simulink model "FYP_Model_ClosedLoop"  (R2014b)
settings: Solver=ode3  StartTime=0.0  StopTime=4  FixedStep=0.0001  MaxStep=0.00001  MinStep=0.00002  RelTol=1e-3
values from neighbouring files (symbols this model uses):
  C = 2.2389314028e-09    [Example_Data.mat]    (also in calculate_constants.m = sqrt(I*K)/Q)
  Capacitance = [1.60057592274e-13 1.6356865827e-13 1.66667495448e-13 1.71350652646e-13 1.74939566926e-13 1.79103436846e-13 1.83468868499e-13 1.88053142462e-13 1.92872426544e-13 1.97945050457e-13 2.03290835825e-13 2.08663004534e-13 ... (161 elements, 1x161)]    [Example_Data.mat]    (also in SC_Transformation.m = E*(l*1e-6)*num_of_gaps)
  I = 2.138022e-10    [Example_Data.mat]    (also in calculate_constants.m = (1/12)*m*w*w)
  K = 8.44057253633e-05    [Example_Data.mat]    (also in calculate_constants.m = Wn*Wn*I)
  theta = [-7.61408173959 -7.51775010326 -7.42143983606 -7.32515065184 -7.22888226498 -7.13263439042 -7.03640674362 -6.94019904057 -6.84401099779 -6.74784233231 -6.65169276165 -6.55556200382 ... (160 elements, 1x160)]    [Example_Data.mat]    (also in SC_Transformation.m = (asin(x1/3000))*(180/pi))
  theta1 = [-7.66225566077 -7.56591323238 -7.46959231642 -7.37329262644 -7.27701387657 -7.18075578146 -7.08451805631 -6.98830041685 -6.89210257935 -6.79592426056 -6.69976517776 -6.60362504873 ... (161 elements, 1x161)]    [Example_Data.mat]    (also in SC_Transformation.m = (asin(x/3000))*(180/pi))
  TorqueN = [1.05331979874e-12 9.29651153439e-13 1.4049471593e-12 1.07667428419e-12 1.24916097602e-12 1.30962949594e-12 1.37528218875e-12 1.44578522446e-12 1.52178717406e-12 1.6037356104e-12 1.6116506126e-12 1.87151628256e-12 ... (160 elements, 1x160)]    [Example_Data.mat]    (also in SC_Transformation.m = Torque/(V*V))
  V = 60    [Example_Data.mat]    (also in SC_Transformation.m = 30; Simulink_Iterate.m = V_array(i))
libraries: simulink x7, simulink_extras x1
settings Model: Creator=Kishan  LastModifiedBy=Kishan
settings DataIOCC: SaveFormat=StructureWithTime  SaveOutput=off  ReturnWorkspaceOutputsName=yout

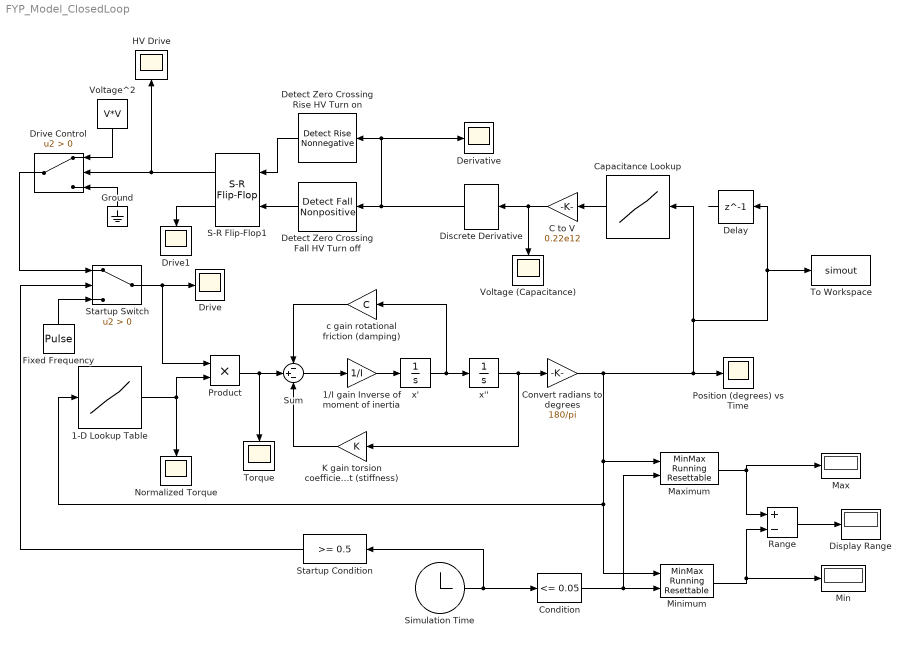
== system FYP_Model_ClosedLoop ==
  1-D Lookup Table : Lookup_n-D  NumberOfTableDimensions=1  BreakpointsForDimension1=theta  IndexSearchMethod=Linear search  Table=TorqueN  InternalRulePriority=Speed  RndMeth=Simplest  InputSameDT=on
  1/I gain Inverse of moment of inertia : Gain  Gain=1/I
  C to V : Gain  Gain=0.22e12
  Capacitance Lookup : Lookup_n-D  NumberOfTableDimensions=1  BreakpointsForDimension1=theta1  IndexSearchMethod=Linear search  Table=Capacitance  InternalRulePriority=Speed  RndMeth=Simplest  InputSameDT=on
  Condition : simulink/Logic and Bit Operations/Compare To Constant  relop=<=  const=0.05  OutDataTypeStr=boolean
  Convert radians to degrees : Gain  Gain=180/pi
  Delay : Delay  DelayLength=1  InitialCondition=0
  Derivative : Scope
      settings: TimeRange=5  YMin=0  YMax=10  SaveName=ScopeData6
  Detect Zero Crossing Fall HV Turn off : simulink/Logic and Bit Operations/Detect Fall Nonpositive  vinit=0  InputProcessing=Inherited  OutDataTypeStr=boolean
  Detect Zero Crossing Rise HV Turn on : simulink/Logic and Bit Operations/Detect Rise Nonnegative  vinit=0  InputProcessing=Inherited  OutDataTypeStr=boolean
  Discrete Derivative : simulink/Discrete/Discrete Derivative  gainval=1.0  ICPrevScaledInput=0.1  InputProcessing=Inherited  OutMin=[]  OutMax=[]  OutDataType=fixdt(1, 16)  OutScaling=2^-10  DoSatur=off
  Display Range : Display
  Drive : Scope
      settings: TimeRange=4  YMin=4.99210822998873  YMax=16.99210822998873  SaveName=ScopeData4
  Drive Control : Switch  Criteria=u2 > Threshold
  Drive1 : Scope
      settings: TimeRange=4  YMin=4.99210822998873  YMax=16.99210822998873  SaveName=ScopeData2
  Fixed Frequency : DiscretePulseGenerator  PulseType=Time based  Amplitude=V*V  Period=0.022  PulseWidth=50  SampleTime=0.0025
  Ground : Ground
  HV Drive : Scope
      settings: TimeRange=3  YMin=0  YMax=1  SaveName=ScopeData11
  K gain torsion coefficient (stiffness) : Gain  Gain=K
  Max : Display
  Maximum : simulink/Math Operations/MinMax Running Resettable  Function=max  vinit=0.0
  Min : Display
  Minimum : simulink/Math Operations/MinMax Running Resettable  Function=min  vinit=10
  Normalized Torque : Scope
      settings: TimeRange=0.009043223963749458  YMin=0  YMax=1
  Position (degrees) vs Time : Scope
      settings: TimeRange=4  YMin=-0.15  YMax=0.15
  Product : Product
  Range : Sum  Inputs=+-
  S-R Flip-Flop1 : simulink_extras/Flip Flops/S-R Flip-Flop  initial_condition=0
  Simulation Time : Clock
  Startup Condition : simulink/Logic and Bit Operations/Compare To Constant  relop=>=  const=0.5  OutDataTypeStr=uint8
  Startup Switch : Switch  Criteria=u2 > Threshold
  Sum : Sum  Inputs=-+-
  To Workspace : ToWorkspace  VariableName=simout  SaveFormat=Structure With Time  SampleTime=-1
  Torque : Scope
      settings: TimeRange=0.009043223963749458  YMin=0  YMax=1  SaveName=ScopeData3
  Voltage (Capacitance) : Scope
      settings: TimeRange=5  YMin=0  YMax=10  SaveName=ScopeData5
  Voltage^2 : Constant  Value=V*V
  c gain rotational friction (damping) : Gain  Gain=C
  x' : Integrator
  x'' : Integrator
  wires:
  x'/1 -> x''/1, c gain rotational friction (damping)/1
  1/I gain Inverse of moment of inertia/1 -> x'/1
  Sum/1 -> 1/I gain Inverse of moment of inertia/1
  K gain torsion coefficient (stiffness)/1 -> Sum/3
  c gain rotational friction (damping)/1 -> Sum/1
  1-D Lookup Table/1 -> Product/2, Normalized Torque/1
  Product/1 -> Torque/1, Sum/2
  x''/1 -> Convert radians to degrees/1, K gain torsion coefficient (stiffness)/1
  Minimum/1 -> Min/1, Range/2
  Maximum/1 -> Max/1, Range/1
  Range/1 -> Display Range/1
  Simulation Time/1 -> Startup Condition/1, Condition/1
  Condition/1 -> Maximum/2, Minimum/2
  Voltage^2/1 -> Drive Control/1
  Ground/1 -> Drive Control/3
  Fixed Frequency/1 -> Startup Switch/3
  Startup Switch/1 -> Drive/1, Product/1
  Drive Control/1 -> Startup Switch/1
  Startup Condition/1 -> Startup Switch/2
  Detect Zero Crossing Rise HV Turn on/1 -> S-R Flip-Flop1/1
  Detect Zero Crossing Fall HV Turn off/1 -> S-R Flip-Flop1/2
  C to V/1 -> Discrete Derivative/1, Voltage (Capacitance)/1
  S-R Flip-Flop1/1 -> Drive Control/2, HV Drive/1
  Capacitance Lookup/1 -> C to V/1
  Discrete Derivative/1 -> Detect Zero Crossing Fall HV Turn off/1, Derivative/1, Detect Zero Crossing Rise HV Turn on/1
  S-R Flip-Flop1/2 -> Drive1/1
  Convert radians to degrees/1 -> Capacitance Lookup/1, Delay/1, To Workspace/1, Position (degrees) vs Time/1, Maximum/1, Minimum/1, 1-D Lookup Table/1
  Delay/1 -> ?
